simulink model "pll06"  (Simulink 8.1)
settings: Solver=ode45  StartTime=0.0  StopTime=2  MaxStep=0.00002  RelTol=1e-3
libraries: commsynccomp2 x1, dsparch4 x1, simulink x1
settings Model: Creator=my88899  LastModifiedBy=my88899
settings DataIOCC: SignalLoggingSaveFormat=Dataset
settings OptimizationCC: ExpressionDepthLimit=128
settings DebuggingCC: FcnCallInpInsideContextMsg=EnableAllAsError
settings GRTTargetCC: CombineOutputUpdateFcns=on  GRTInterface=off

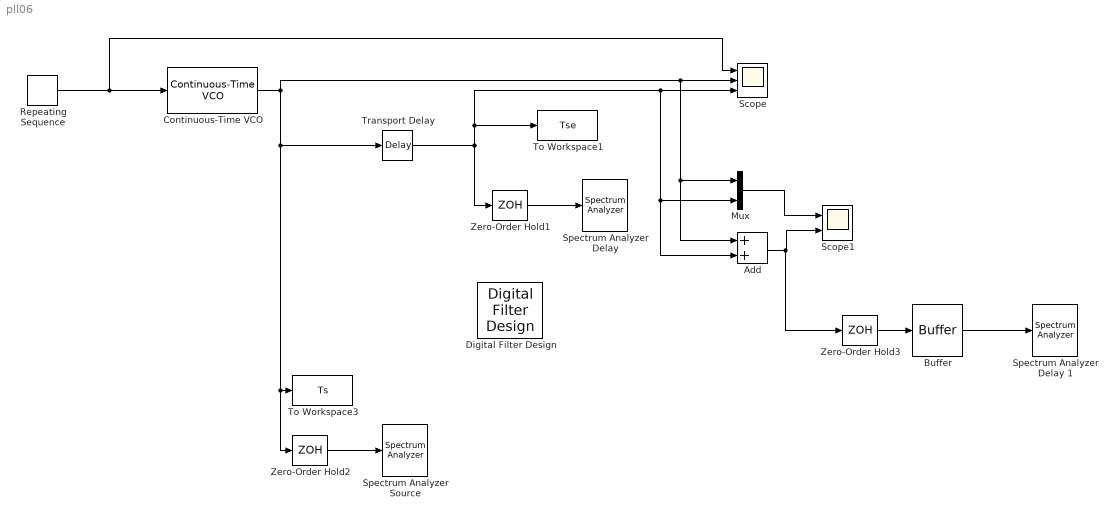
== system pll06 ==
  Add : Sum
  Buffer : Buffer  N=1000  TreatMby1Signals=One channel
  Continuous-Time VCO : commsynccomp2/Continuous-Time VCO  Ac=5  Fc=1000  Kc=1000  Ph=0
  Digital Filter Design : dsparch4/Digital Filter Design  mwdsp_browser_bugfix_var=off
  Mux : Mux  Inputs=2
  Repeating Sequence : simulink/Sources/Repeating Sequence  rep_seq_t=[0 1]  rep_seq_y=[0 4]
  Scope : Scope  NumInputPorts=3
      settings: TimeRange=0.1038961038961048  YMin=5.645~-5~-5  YMax=5.7~5~5  MaxDataPoints=100000
  Scope1 : Scope  NumInputPorts=2
      settings: TimeRange=0.1038961038961048  YMin=-10~-15  YMax=10~15  MaxDataPoints=100000
  "Spectrum Analyzer Delay " : SpectrumAnalyzer
      settings: CopyFcn=scopeextensions.ScopeBlock.callback(gcbh, 'onBlockCopy', gcbh);  DeleteFcn=scopeextensions.ScopeBlock.callback(gcbh, 'onBlockDelete');  PreSaveFcn=scopeextensions.ScopeBlock.callback(gcbh, 'onModelSave');  NameChangeFcn=scopeextensions.ScopeBlock.callback(gcbh, 'onBlockRename');  CloseFcn=scopeextensions.ScopeBlock.callback(gcbh, 'onBlockClose');  PreDeleteFcn=scopeextensions.ScopeBlock.callback(gcbh, 'onBlockPreDelete');
  Spectrum Analyzer Delay 1 : SpectrumAnalyzer
      settings: CopyFcn=scopeextensions.ScopeBlock.callback(gcbh, 'onBlockCopy', gcbh);  DeleteFcn=scopeextensions.ScopeBlock.callback(gcbh, 'onBlockDelete');  PreSaveFcn=scopeextensions.ScopeBlock.callback(gcbh, 'onModelSave');  NameChangeFcn=scopeextensions.ScopeBlock.callback(gcbh, 'onBlockRename');  CloseFcn=scopeextensions.ScopeBlock.callback(gcbh, 'onBlockClose');  PreDeleteFcn=scopeextensions.ScopeBlock.callback(gcbh, 'onBlockPreDelete');
  "Spectrum Analyzer Source " : SpectrumAnalyzer
      settings: CopyFcn=scopeextensions.ScopeBlock.callback(gcbh, 'onBlockCopy', gcbh);  DeleteFcn=scopeextensions.ScopeBlock.callback(gcbh, 'onBlockDelete');  PreSaveFcn=scopeextensions.ScopeBlock.callback(gcbh, 'onModelSave');  NameChangeFcn=scopeextensions.ScopeBlock.callback(gcbh, 'onBlockRename');  CloseFcn=scopeextensions.ScopeBlock.callback(gcbh, 'onBlockClose');  PreDeleteFcn=scopeextensions.ScopeBlock.callback(gcbh, 'onBlockPreDelete');
  To Workspace1 : ToWorkspace  VariableName=Tse  SampleTime=-1  SaveFormat=Timeseries
  To Workspace3 : ToWorkspace  VariableName=Ts  SampleTime=-1  SaveFormat=Timeseries
  Transport Delay : TransportDelay  DelayTime=0.12
  Zero-Order Hold1 : ZeroOrderHold  SampleTime=0.001
  Zero-Order Hold2 : ZeroOrderHold  SampleTime=0.001
  Zero-Order Hold3 : ZeroOrderHold  SampleTime=0.001
  wires:
  Repeating Sequence/1 -> Scope/1, Continuous-Time VCO/1
  Zero-Order Hold1/1 -> "Spectrum Analyzer Delay "/1
  Zero-Order Hold2/1 -> "Spectrum Analyzer Source "/1
  Continuous-Time VCO/1 -> Zero-Order Hold2/1, To Workspace3/1, Transport Delay/1, Add/1, Mux/1, Scope/2
  Transport Delay/1 -> Add/2, Mux/2, Scope/3, To Workspace1/1, Zero-Order Hold1/1
  Mux/1 -> Scope1/1
  Add/1 -> Zero-Order Hold3/1, Scope1/2
  Buffer/1 -> Spectrum Analyzer Delay 1/1
  Zero-Order Hold3/1 -> Buffer/1
